simulink model "untitled1"  (R2020b)
settings: Solver=VariableStepAuto  StartTime=0.0  StopTime=120  RelTol=1e-3
model workspace (MAT data in the model file):
  B = Simulink.Parameter
  B.Value = 50
  B.DataType = 'auto'
  B.Dimensions = [1 1]
  Kd = Simulink.Parameter
  Kd.Value = 484.0516
  Kd.DataType = 'auto'
  Kd.Dimensions = [1 1]
  Ki = Simulink.Parameter
  Ki.Value = 83.0917
  Ki.DataType = 'auto'
  Ki.Dimensions = [1 1]
  Kp = Simulink.Parameter
  Kp.Value = 495.0505
  Kp.DataType = 'auto'
  Kp.Dimensions = [1 1]
  M = Simulink.Parameter
  M.Value = 1000
  M.DataType = 'auto'
  M.Dimensions = [1 1]
settings Model: Creator=varunraj  LastModifiedBy=varunraj

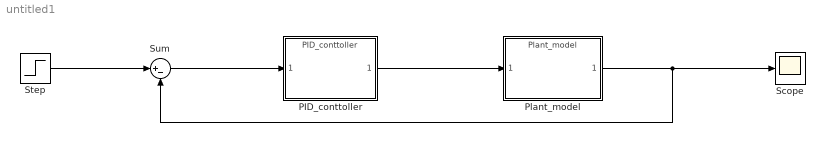
== system untitled1 ==
  PID_conttoller : ModelReference  ModelNameDialog=PID_conttoller  SimulationMode=Normal  ModelReferenceVersion=1.1
  Plant_model : ModelReference  ModelNameDialog=Plant_model  SimulationMode=Normal  ModelReferenceVersion=1.1
  Scope : Scope
  Step : Step  After=10  SampleTime=0
  Sum : Sum  Inputs=|+-
  wires:
  Step/1 -> Sum/1
  Sum/1 -> PID_conttoller/1
  Plant_model/1 -> Sum/2, Scope/1
  PID_conttoller/1 -> Plant_model/1
